simulink library "Humanoid_RL_Lib"  (R2025b)
settings: Solver=VariableStepAuto  StartTime=0.0  StopTime=10.0  RelTol=1e-3
undefined symbols (not defined in the file or in its folder): params
libraries: simulink x7
settings Model: Creator=The MathWorks, Inc.  LastModifiedBy=jolson
settings SolverCC: AlgebraicLoopSolver=TrustRegion
settings DebuggingCC: UnconnectedInputMsg=warning  UnconnectedOutputMsg=warning  UnconnectedLineMsg=warning
settings ModelReferenceCC: EnableRefExpFcnMdlSchedulingChecks=on
settings RTWCC: GPUComputeCapability=3.5  DLArmComputeVersion=19.05

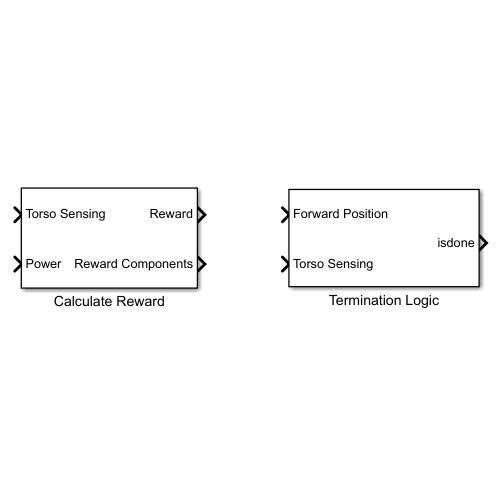
[thumbnail: Simulink's stored preview of the top-level diagram]
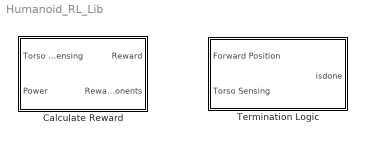
== system Humanoid_RL_Lib ==
  Calculate Reward : Subsystem  mask{forwardReward=params.reward.forwardRewardWeight, timestepReward=params.reward.timestepRewardWeight, powerPenalty=params.reward.powerPenaltyWeight, verticalPenalty=params.reward.verticalPenaltyWeight, lateralPenalty=params.reward.lateralPenaltyWeight}
      mask prompts: forwardReward "Forward velcoity reward scaling"; timestepReward "Timestep reward scaling"; powerPenalty "Power penalty scaling"; verticalPenalty "Vertical displacement penalty scaling"; lateralPenalty "Lateral displacement penalty scaling"
  Termination Logic : Subsystem  mask{verticalStop=params.stoppingCriteria.heightChange, lateralStop=params.stoppingCriteria.lateral, angularStop=params.stoppingCriteria.angle, timeoutTime=params.stoppingCriteria.timeoutTime, timeoutDistance=params.stoppingCriteria.timeoutDistance}
      mask prompts: verticalStop "Vertical Displacement Stopping Criteria (m)"; lateralStop "Lateral Displacement Stopping Criteria (m)"; angularStop "Rotation Stopping Criteria (deg)"; timeoutTime "Timeout Time"; timeoutDistance "Timeout Distance"

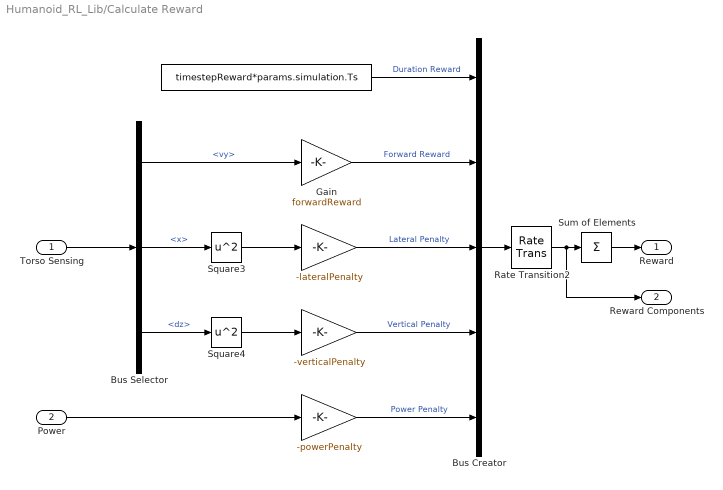
== system Humanoid_RL_Lib/Calculate Reward ==
  Torso Sensing : Inport
  Power : Inport  Port=2
  " " : Gain  Gain=-lateralPenalty
  "     " : Gain  Gain=-verticalPenalty
  "                    " : Gain  Gain=-powerPenalty
  "                       " : Constant  Value=timestepReward*params.simulation.Ts
  Bus Creator : BusCreator  Inputs=5
  Bus Selector : BusSelector  OutputSignals=signal2.vy,signal2.x,signal2.dz
  Gain : Gain  Gain=forwardReward
  Rate Transition2 : RateTransition  OutPortSampleTime=params.simulation.Ts
  Square3 : Math  Operator=square  SignedPower=on
  Square4 : Math  Operator=square  SignedPower=on
  Sum of Elements : Sum  Inputs=+
  Reward : Outport  VectorParamsAs1DForOutWhenUnconnected=off
  Reward Components : Outport  Port=2  VectorParamsAs1DForOutWhenUnconnected=off
  wires:
  Torso Sensing/1 -> Bus Selector/1
  Power/1 -> "                    "/1
  Square4/1 -> "     "/1
  Bus Selector/3 -> Square4/1  "<dz>"
  Square3/1 -> " "/1
  Bus Selector/2 -> Square3/1  "<x>"
  Sum of Elements/1 -> Reward/1
  " "/1 -> Bus Creator/3  "Lateral Penalty"
  "                    "/1 -> Bus Creator/5  "Power Penalty"
  "                       "/1 -> Bus Creator/1  "Duration Reward"
  Bus Selector/1 -> Gain/1  "<vy>"
  Gain/1 -> Bus Creator/2  "Forward Reward"
  "     "/1 -> Bus Creator/4  "Vertical Penalty"
  Bus Creator/1 -> Rate Transition2/1
  Rate Transition2/1 -> Reward Components/1, Sum of Elements/1

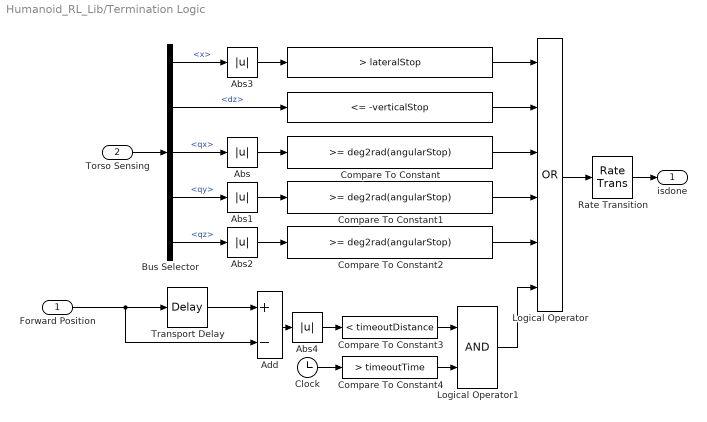
== system Humanoid_RL_Lib/Termination Logic ==
  Forward Position : Inport
  Torso Sensing : Inport  Port=2
  " " : simulink/Logic and Bit Operations/Compare To Constant  relop=<=  const=-verticalStop  OutDataTypeStr=boolean  ZeroCross=off
  "             " : simulink/Logic and Bit Operations/Compare To Constant  relop=>  const=lateralStop  OutDataTypeStr=boolean
  Abs{,1..3} (4 alike) : Abs  ZeroCross=off  SaturateOnIntegerOverflow=off
  Abs4 : Abs  SaturateOnIntegerOverflow=off
  Add : Sum  Inputs=+-
  Bus Selector : BusSelector  OutputSignals=signal2.x,signal2.dz,signal1.qx,signal1.qy,signal1.qz
  Clock : Clock
  Compare To Constant : simulink/Logic and Bit Operations/Compare To Constant  relop=>=  const=deg2rad(angularStop)  OutDataTypeStr=boolean  ZeroCross=off
  Compare To Constant1 : simulink/Logic and Bit Operations/Compare To Constant  relop=>=  const=deg2rad(angularStop)  OutDataTypeStr=boolean  ZeroCross=off
  Compare To Constant2 : simulink/Logic and Bit Operations/Compare To Constant  relop=>=  const=deg2rad(angularStop)  OutDataTypeStr=boolean  ZeroCross=off
  Compare To Constant3 : simulink/Logic and Bit Operations/Compare To Constant  relop=<  const=timeoutDistance  OutDataTypeStr=boolean
  Compare To Constant4 : simulink/Logic and Bit Operations/Compare To Constant  relop=>  const=timeoutTime  OutDataTypeStr=boolean
  Logical Operator : Logic  Operator=OR  Inputs=6  AllPortsSameDT=off  OutDataTypeStr=boolean
  Logical Operator1 : Logic  AllPortsSameDT=off  OutDataTypeStr=boolean
  Rate Transition : RateTransition  OutPortSampleTime=params.simulation.Ts
  Transport Delay : TransportDelay  DelayTime=timeoutTime  BufferSize=8192
  isdone : Outport  VectorParamsAs1DForOutWhenUnconnected=off
  wires:
  Bus Selector/2 -> " "/1  "<dz>"
  Torso Sensing/1 -> Bus Selector/1
  " "/1 -> Logical Operator/2
  Bus Selector/3 -> Abs/1  "<qx>"
  Bus Selector/4 -> Abs1/1  "<qy>"
  Compare To Constant/1 -> Logical Operator/3
  Abs/1 -> Compare To Constant/1
  Abs1/1 -> Compare To Constant1/1
  Logical Operator/1 -> Rate Transition/1
  Abs3/1 -> "             "/1
  Bus Selector/1 -> Abs3/1  "<x>"
  "             "/1 -> Logical Operator/1
  Abs2/1 -> Compare To Constant2/1
  Bus Selector/5 -> Abs2/1  "<qz>"
  Compare To Constant2/1 -> Logical Operator/5
  Compare To Constant1/1 -> Logical Operator/4
  Rate Transition/1 -> isdone/1
  Forward Position/1 -> Add/2, Transport Delay/1
  Transport Delay/1 -> Add/1
  Add/1 -> Abs4/1
  Abs4/1 -> Compare To Constant3/1
  Clock/1 -> Compare To Constant4/1
  Logical Operator1/1 -> Logical Operator/6
  Compare To Constant3/1 -> Logical Operator1/1
  Compare To Constant4/1 -> Logical Operator1/2
